simulink subsystem "Heat_Balance_Equation"  (R2023b)
settings: Solver=VariableStepAuto  StartTime=0.0  StopTime=10.0  RelTol=1e-3
settings Model: Creator=gio  LastModifiedBy=gio

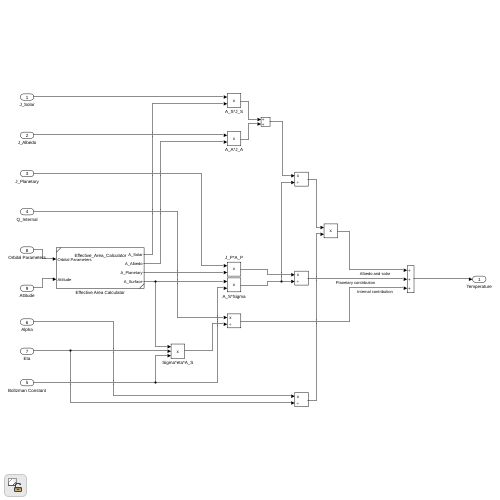
[thumbnail: Simulink's stored preview of the top-level diagram]
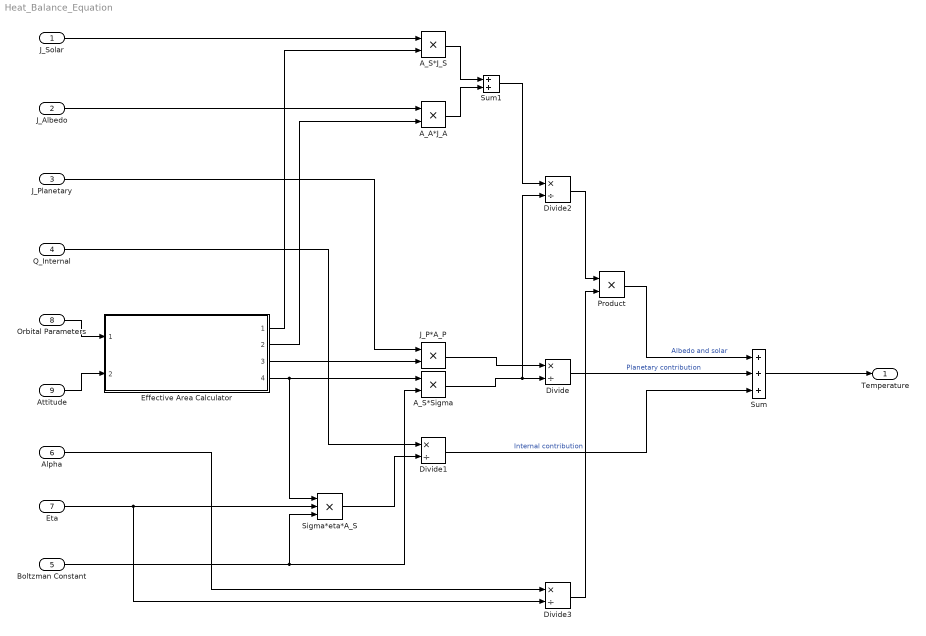
== system Heat_Balance_Equation ==
  J_Solar : Inport
  J_Albedo : Inport  Port=2
  J_Planetary : Inport  Port=3
  Q_Internal : Inport  Port=4
  Boltzman Constant : Inport  Port=5
  Alpha : Inport  Port=6
  Eta : Inport  Port=7
  Orbital Parameters : Inport  Port=8
  Attitude : Inport  Port=9
  A_A*J_A : Product
  A_S*J_S : Product
  A_S*Sigma : Product
  Divide{,1..3} (4 alike) : Product  Inputs=*/
  Effective Area Calculator : Subsystem  ReferencedSubsystem=Effective_Area_Calculator
  J_P*A_P : Product
  Product : Product
  Sigma*eta*A_S : Product  Inputs=3
  Sum : Sum  Inputs=+++
  Sum1 : Sum
  Temperature : Outport
  wires:
  Attitude/1 -> Effective Area Calculator/2
  Orbital Parameters/1 -> Effective Area Calculator/1
  J_P*A_P/1 -> Divide/1
  A_S*Sigma/1 -> Divide/2, Divide2/2
  Boltzman Constant/1 -> A_S*Sigma/2, Sigma*eta*A_S/3
  J_Planetary/1 -> J_P*A_P/1
  Effective Area Calculator/3 -> J_P*A_P/2
  Effective Area Calculator/4 -> A_S*Sigma/1, Sigma*eta*A_S/1
  Divide/1 -> Sum/2  "Planetary contribution"
  Eta/1 -> Sigma*eta*A_S/2, Divide3/2
  Q_Internal/1 -> Divide1/1
  Sigma*eta*A_S/1 -> Divide1/2
  Divide1/1 -> Sum/3  "Internal contribution"
  J_Solar/1 -> A_S*J_S/1
  J_Albedo/1 -> A_A*J_A/1
  Effective Area Calculator/1 -> A_S*J_S/2
  Effective Area Calculator/2 -> A_A*J_A/2
  A_S*J_S/1 -> Sum1/1
  A_A*J_A/1 -> Sum1/2
  Sum/1 -> Temperature/1
  Sum1/1 -> Divide2/1
  Alpha/1 -> Divide3/1
  Divide2/1 -> Product/1
  Divide3/1 -> Product/2
  Product/1 -> Sum/1  "Albedo and solar"
